simulink model "chap1_2"  (R2023b)
settings: Solver=ode45  StartTime=0.0  StopTime=10.0  RelTol=1e-3
settings Model: Creator=CorgiQvm  LastModifiedBy=CorgiQvm
settings DataIOCC: ReturnWorkspaceOutputs=off

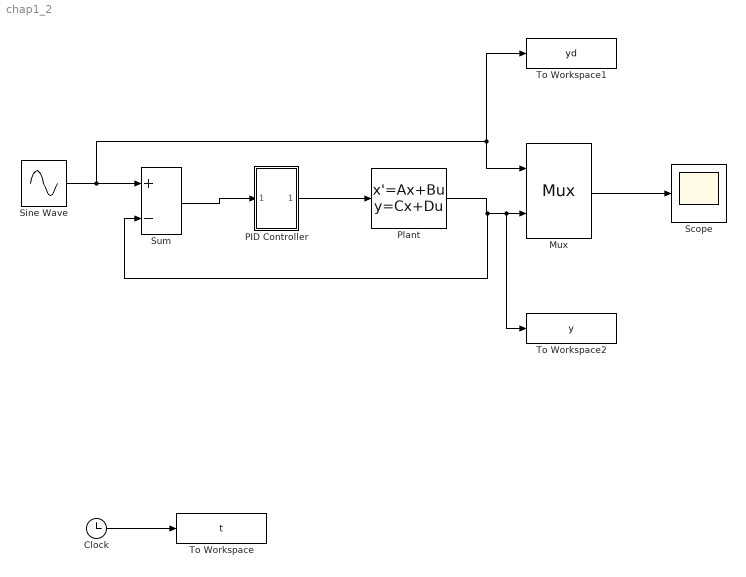
== system chap1_2 ==
  Clock : Clock
  Mux : Mux  Inputs=2
  PID Controller : Subsystem  mask{P=60, I=1, D=3}
      mask prompts: P "Proportional"; I "Integral"; D "Derivative"
      mask DialogControl ParameterGroupVar Prompt: 参数
      mask Display: disp('PID');
  Plant : StateSpace  A=[0 1;0 -25]  B=[0;133]  C=[1 0]  D=zeros(1)  InitialCondition=0
  Scope : Scope
  Sine Wave : Sin  Frequency=0.20*2*pi  SampleTime=0
  Sum : Sum  Inputs=+-  InputSameDT=on  SaturateOnIntegerOverflow=on  OutDataTypeStr=Inherit: Same as first input
  To Workspace : ToWorkspace  VariableName=t  SampleTime=-1
  To Workspace1 : ToWorkspace  VariableName=yd  SampleTime=-1
  To Workspace2 : ToWorkspace  VariableName=y  SampleTime=-1
  wires:
  Sine Wave/1 -> Mux/1, To Workspace1/1, Sum/1
  Sum/1 -> PID Controller/1(In1)
  PID Controller/1(Out1) -> Plant/1
  Plant/1 -> Sum/2, To Workspace2/1, Mux/2
  Mux/1 -> Scope/1
  Clock/1 -> To Workspace/1

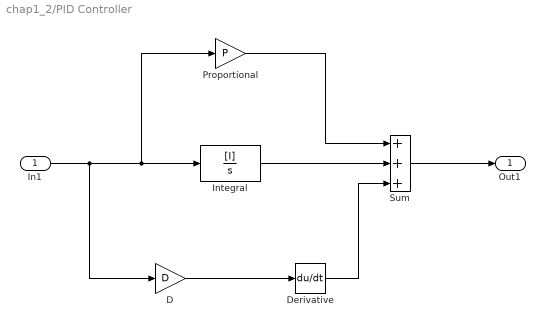
== system chap1_2/PID Controller ==
  In1 : Inport
  D : Gain  Gain=D  SaturateOnIntegerOverflow=on  OutDataTypeStr=Inherit: Same as input  ParamDataTypeStr=Inherit: Same as input
  Derivative : Derivative
  Integral : TransferFcn  Numerator=[I]  Denominator=[1 0]
  Proportional : Gain  Gain=P  SaturateOnIntegerOverflow=on  OutDataTypeStr=Inherit: Same as input  ParamDataTypeStr=Inherit: Same as input
  Sum : Sum  Inputs=+++  InputSameDT=on  SaturateOnIntegerOverflow=on  OutDataTypeStr=Inherit: Same as first input
  Out1 : Outport
  wires:
  D/1 -> Derivative/1
  Integral/1 -> Sum/2
  Proportional/1 -> Sum/1
  In1/1 -> D/1, Proportional/1, Integral/1
  Sum/1 -> Out1/1
  Derivative/1 -> Sum/3
